simulink model "Subsistema_electromagnetico"  (R2021a)
settings: Solver=VariableStepAuto  StartTime=0.0  StopTime=10.0  RelTol=1e-3
undefined symbols (not defined in the file): lambda_m, Ld, Lls, Lq, Pp, Rs
settings Model: Creator=fhlla  LastModifiedBy=fhlla

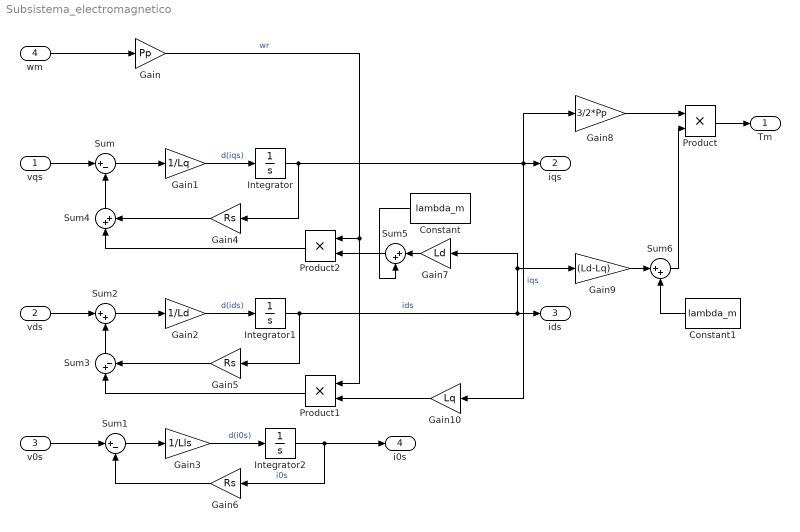
== system Subsistema_electromagnetico ==
  vqs : Inport
  vds : Inport  Port=2
  v0s : Inport  Port=3
  wm : Inport  Port=4
  Constant : Constant  Value=lambda_m
  Constant1 : Constant  Value=lambda_m
  Gain : Gain  Gain=Pp
  Gain1 : Gain  Gain=1/Lq
  Gain10 : Gain  Gain=Lq
  Gain2 : Gain  Gain=1/Ld
  Gain3 : Gain  Gain=1/Lls
  Gain4 : Gain  Gain=Rs
  Gain5 : Gain  Gain=Rs
  Gain6 : Gain  Gain=Rs
  Gain7 : Gain  Gain=Ld
  Gain8 : Gain  Gain=3/2*Pp
  Gain9 : Gain  Gain=(Ld-Lq)
  Integrator : Integrator
  Integrator1 : Integrator
  Integrator2 : Integrator
  Product : Product
  Product1 : Product
  Product2 : Product
  Sum : Sum  Inputs=|+-
  Sum1 : Sum  Inputs=|+-
  Sum{2,4..6} (4 alike) : Sum  Inputs=|++
  Sum3 : Sum  Inputs=|+-
  Tm : Outport
  iqs : Outport  Port=2
  ids : Outport  Port=3
  i0s : Outport  Port=4
  wires:
  vds/1 -> Sum2/1
  Sum3/1 -> Sum2/2
  Sum2/1 -> Gain2/1
  Gain2/1 -> Integrator1/1  "d(ids)"
  Gain5/1 -> Sum3/2
  Product1/1 -> Sum3/1
  Integrator1/1 -> Gain5/1, Gain9/1, Gain7/1, ids/1  "ids"
  wm/1 -> Gain/1
  Gain/1 -> Product2/1, Product1/1  "wr"
  vqs/1 -> Sum/1
  Sum/1 -> Gain1/1
  Gain4/1 -> Sum4/2
  Sum4/1 -> Sum/2
  Gain1/1 -> Integrator/1  "d(iqs)"
  Integrator/1 -> Gain4/1, Gain10/1, Gain8/1, iqs/1  "iqs"
  Product2/1 -> Sum4/1
  Sum5/1 -> Product2/2
  Constant/1 -> Sum5/2
  Gain7/1 -> Sum5/1
  Gain10/1 -> Product1/2
  Gain8/1 -> Product/1
  Product/1 -> Tm/1
  Gain9/1 -> Sum6/1
  Sum6/1 -> Product/2
  Constant1/1 -> Sum6/2
  v0s/1 -> Sum1/1
  Sum1/1 -> Gain3/1
  Gain3/1 -> Integrator2/1  "d(i0s)"
  Integrator2/1 -> Gain6/1, i0s/1  "i0s"
  Gain6/1 -> Sum1/2
